simulink model "passivefilter_final"  (R2015a)
settings: Solver=ode45  StartTime=0.0  StopTime=0.1  RelTol=1e-3
libraries: powerlib x12
settings Model: Creator=gautam  LastModifiedBy=gautam

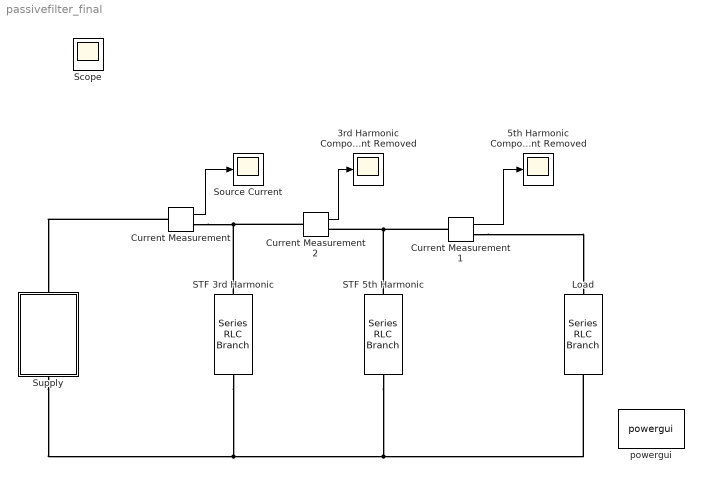
== system passivefilter_final ==
  3rd Harmonic Component Removed : Scope
      settings: SaveName=Filtered_Current1
  5th Harmonic Component Removed : Scope
      settings: SaveName=Filtered_Current2
  Current Measurement : powerlib/Measurements/Current Measurement  PhasorSimulation=off  OutputType=Complex  PSBequivalent=0
  Current Measurement1 : powerlib/Measurements/Current Measurement  PhasorSimulation=off  OutputType=Complex  PSBequivalent=0
  Current Measurement2 : powerlib/Measurements/Current Measurement  PhasorSimulation=off  OutputType=Complex  PSBequivalent=0
  Load : powerlib/Elements/Series RLC Branch  LConnTagsString=__new0  RConnTagsString=__new0  BranchType=R  Resistance=1  Inductance=1e-3  SetiL0=off  InitialCurrent=0  Capacitance=1e-6  Setx0=off  InitialVoltage=0  Measurements=Branch voltage and current
  STF 3rd Harmonic : powerlib/Elements/Series RLC Branch  LConnTagsString=__new0  RConnTagsString=__new0  BranchType=RLC  Resistance=0.0027741142474339464  Inductance=0.000147199  SetiL0=off  InitialCurrent=0  Capacitance=8e-3  Setx0=off  InitialVoltage=0  Measurements=None
  STF 5th Harmonic : powerlib/Elements/Series RLC Branch  LConnTagsString=__new0  RConnTagsString=__new0  BranchType=RLC  Resistance=0.0016644685484603675  Inductance=0.000052991  SetiL0=off  InitialCurrent=0  Capacitance=0.007650969  Setx0=off  InitialVoltage=0  Measurements=None
  Source Current : Scope
      settings: SaveName=Source_Current
  Supply : Subsystem
  powergui : powerlib/powergui  Priority=1  SimulationMode=Continuous  SolverType=Tustin/Backward Euler (TBE)  SampleTime=50e-6  frequency=60  SPID=off  DisableSnubberDevices=off  DisableRonSwitches=off  DisableVfSwitches=off  SwTol=0  DisplayEquations=off  Interpol=off  methode=off  Ts=100  FunctionMessages=off  echomessages=off  HookPort=off  EnableUseOfTLC=off  x0status=blocks  frequencyindice=50  Pbase=100e6  ErrMax=1e-4  Iterations=50  UnitsV=kV  UnitsW=MW  buscounter=0  RestoreLinks=warning  ResistiveCurrentMeasurement=off  Frange=[0:2:500]  Ylog=off  Xlog=on  ShowGrid=off  save=off  variable=ZData  structure=Filtered_Current2  ZoomFFT=off  StartTime=0.0  cycles=1  DisplayStyle=1  fundamental=50  FreqAxis=on  MaxFrequency=500  frequencyindicesteady=1  RmsSteady=1  display=off
  Scope : Scope
  wires:
  Current Measurement2/1 -> 3rd Harmonic Component Removed/1
  Current Measurement1/1 -> 5th Harmonic Component Removed/1
  Current Measurement/1 -> Source Current/1
  connections:
  Supply/LConn1 -- STF 3rd Harmonic/RConn1 -- STF 5th Harmonic/RConn1 -- Load/RConn1
  Current Measurement/RConn1 -- STF 3rd Harmonic/LConn1 -- Current Measurement2/LConn1
  Current Measurement1/LConn1 -- STF 5th Harmonic/LConn1 -- Current Measurement2/RConn1
  Current Measurement1/RConn1 -- Load/LConn1
  Current Measurement/LConn1 -- Supply/RConn1

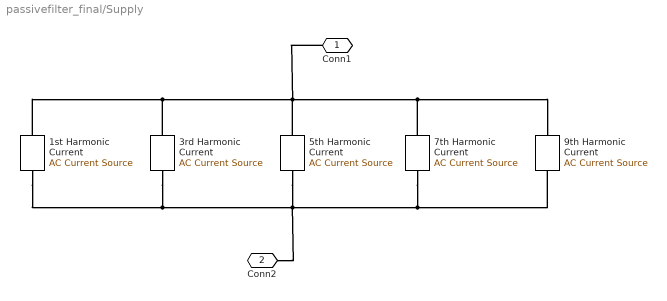
== system passivefilter_final/Supply ==
  1st Harmonic Current : powerlib/Electrical Sources/AC Current Source  Amplitude=10  Phase=0  Frequency=50  SampleTime=0  Measurements=Current
  3rd Harmonic Current : powerlib/Electrical Sources/AC Current Source  Amplitude=8.4  Phase=0  Frequency=150  SampleTime=0  Measurements=Current
  5th Harmonic Current : powerlib/Electrical Sources/AC Current Source  Amplitude=6.3  Phase=0  Frequency=250  SampleTime=0  Measurements=Current
  7th Harmonic Current : powerlib/Electrical Sources/AC Current Source  Amplitude=3.8  Phase=0  Frequency=350  SampleTime=0  Measurements=Current
  9th Harmonic Current : powerlib/Electrical Sources/AC Current Source  Amplitude=1.6  Phase=0  Frequency=450  SampleTime=0  Measurements=Current
  Conn1 : PMIOPort  Port=1  Side=Right
  Conn2 : PMIOPort  Port=2  Side=Left
  connections:
  1st Harmonic Current/RConn1 -- 3rd Harmonic Current/RConn1 -- Conn1/RConn1 -- 5th Harmonic Current/RConn1 -- 7th Harmonic Current/RConn1 -- 9th Harmonic Current/RConn1
  1st Harmonic Current/LConn1 -- 3rd Harmonic Current/LConn1 -- Conn2/RConn1 -- 5th Harmonic Current/LConn1 -- 9th Harmonic Current/LConn1 -- 7th Harmonic Current/LConn1
